simulink model "Test"  (R2022a)
settings: Solver=VariableStepAuto  StartTime=0.0  StopTime=100  RelTol=1e-3
libraries: fl_lib x1, nesl_utility x1
settings Model: Creator=mateu  LastModifiedBy=mateu

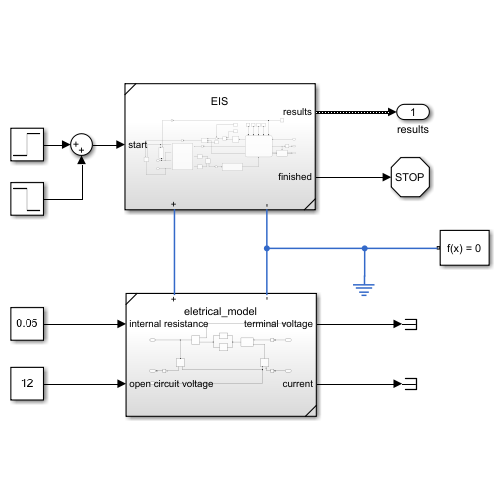
[thumbnail: Simulink's stored preview of the top-level diagram]
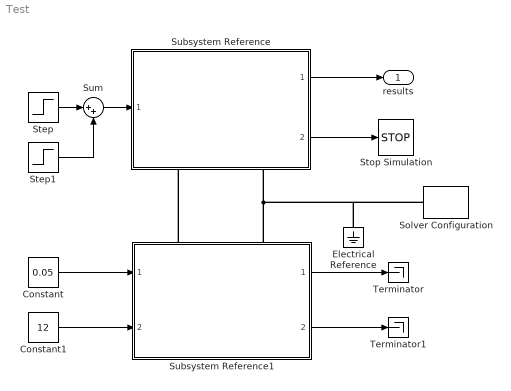
== system Test ==
  Constant : Constant  Value=0.05
  Constant1 : Constant  Value=12
  Electrical Reference : fl_lib/Electrical/Electrical Elements/Electrical Reference
      settings: SourceProductBaseCode=PW,SS,VE
  Solver Configuration : nesl_utility/Solver Configuration  PhysicalDomain=network_engine_domain  SubClassName=solver  LeftPortType=input  RightPortType=generic  Tones=[]  Harmonics=[]  SimulateNoise=off  Profile=off  UseLocalSampling=off  EnableSwitchedLinearOptims=on  FrequencyDomain=off  UseCCode=off  RelTol=0.001  AbsTol=0.001  MinStep=1e-09  ToWorkspace=off  RevertToSquareIcSolve=off  NumHomotopyIterations=100  PhasorMode=off  PhasorModeNumHarmonics=1  IndexReductionMethod=DerivativeReplacement  DoDC=off  ResidualTolerance=1e-09  UseLocalSolver=off  LocalSolverChoice=NE_BACKWARD_EULER_ADVANCER  LocalSolverSampleTime=0.001  DoFixedCost=off  MaxNonlinIter=3  MaxModeIter=2  ComputeImpulses=off  ImpulseIterations=2  LinearAlgebra=auto  LinearAlgebraNumThread=0  EquationFormulation=NE_TIME_EF  DelaysMemoryBudget=1024  AutomaticFiltering=on  FilteringTimeConstant=0.001  PartitionStorageMethod=AS_NEEDED  PartitionMemoryBudget=1024  PartitionMethod=ROBUST
      settings: SourceProductBaseCode=SS,PW,VE
  Step : Step  Time=0.1  SampleTime=0
  Step1 : Step  Time=0.2  After=-1  SampleTime=0
  Stop Simulation : Stop
  Subsystem Reference : Subsystem  ReferencedSubsystem=EIS
      settings: PortSchema="{\"entries\":[{\"content\":{\"sides\":[{\"content\":{\"connectorIds\":[\"In1\"]},\"type\":\"ConnectorPlacement.EquallySpacedRectSide\",\"uuid\":\"b4295795-bb4f-4226-ae08-13ff31e69c7e\"},{\"content\":{\"connectorIds\":[\"Out1\",\"Out2\"],\"side\":\"RIGHT\"},\"type\":\"ConnectorPlacement.EquallySpacedRectSide\",\"uuid\":\"cf500fd2-35e2-47f1-8094-2f89cbc86857\"},{\"content\":{\"connectorIds\":[],\"side\":\"TOP\"},\"type\":\"ConnectorPlacement.EquallySpacedRectSide\",\"uuid\":\"635a65a1-d415-436a-9540-513bae37053e\"},{\"content\":{\"connectorIds\":[\"LConn1\",\"LConn2\"],\"side\":\"BOTTOM\"},\"type\":\"ConnectorPlacement.EquallySpacedRectSide\",\"uuid\":\"4a009bf0-cf28-4e0c-8c34-5f22a3bb1250\"}]},\"type\":\"ConnectorPlacement.EquallySpacedConnector\",\"uuid\":\"170704b4-cdd6-4628-9347-edd0fb851791\"}],\"packageUris\":[\"http://schema.mathworks.com/mf0/Connector/R2020b\"],\"version\":\"1.0\"}"
  Subsystem Reference1 : Subsystem  ReferencedSubsystem=eletrical_model
      settings: PortSchema="{\"entries\":[{\"content\":{\"sides\":[{\"content\":{\"connectorIds\":[\"In1\",\"In2\"]},\"type\":\"ConnectorPlacement.EquallySpacedRectSide\",\"uuid\":\"747fffec-1188-4560-a63f-e796ff73abc9\"},{\"content\":{\"connectorIds\":[\"Out1\",\"Out2\"],\"side\":\"RIGHT\"},\"type\":\"ConnectorPlacement.EquallySpacedRectSide\",\"uuid\":\"c8b2c27b-57f0-426f-8f7f-d4e2bbdef76e\"},{\"content\":{\"connectorIds\":[\"LConn1\",\"LConn2\"],\"side\":\"TOP\"},\"type\":\"ConnectorPlacement.EquallySpacedRectSide\",\"uuid\":\"aa3beff7-3052-4685-a7af-7f3c81e4b1e5\"}]},\"type\":\"ConnectorPlacement.EquallySpacedConnector\",\"uuid\":\"a83fffc3-2d86-4bd9-832d-7e01edf78d97\"}],\"packageUris\":[\"http://schema.mathworks.com/mf0/Connector/R2020b\"],\"version\":\"1.0\"}"
  Sum : Sum  Inputs=|++
  Terminator : Terminator
  Terminator1 : Terminator
  results : Outport
  wires:
  Constant/1 -> Subsystem Reference1/1
  Constant1/1 -> Subsystem Reference1/2
  Subsystem Reference1/1 -> Terminator/1
  Subsystem Reference1/2 -> Terminator1/1
  Step/1 -> Sum/1
  Step1/1 -> Sum/2
  Sum/1 -> Subsystem Reference/1
  Subsystem Reference/1 -> results/1
  Subsystem Reference/2 -> Stop Simulation/1
  connections:
  Subsystem Reference1/LConn1 -- Subsystem Reference/LConn1
  Subsystem Reference1/LConn2 -- Subsystem Reference/LConn2 -- Solver Configuration/RConn1 -- Electrical Reference/LConn1
